simulink model "A17_PID_Lorentzaktuator"  (R2017b)
settings: Solver=ode45  StartTime=0.0  StopTime=15  MaxStep=1e-4  RelTol=1e-3  EnableMultiTasking=on
model workspace (MAT data in the model file):
  CF = 200000
  CR = 10
  KF = 50
  KV = 50
  LM = 0.01
  RM = 4
  Umax = 120
  g = 9.81
  m1 = 1
  m2 = 4
values from neighbouring files (symbols this model uses):
  CD = 1e1    (= 10)    [A14_Konstanten.m]    (also in A17_Konstanten.m = 100; A8_Konstanten.m = 20; A9_Konstanten.m = 0.1)
undefined symbols (not defined in the file or in its folder): sigbuilder_block
libraries: simulink x3
settings Model: Creator=jbaur  LastModifiedBy=jbaur
settings DataIOCC: ExternalInput=X1  SaveFormat=StructureWithTime  InspectSignalLogs=on  SignalLoggingName=sigsOut
settings OptimizationCC: ExpressionDepthLimit=2147483647  InitFltsAndDblsToZero=on  LifeSpan=inf
settings DebuggingCC: SaveWithParameterizedLinksMsg=none  SignalResolutionControl=TryResolveAllWithWarning  MultiTaskDSMMsg=warning  MultiTaskCondExecSysMsg=none  StateNameClashWarn=warning  SFUnexpectedBacktrackingDiag=warning  SFNoUnconditionalDefaultTransitionDiag=warning  SFExecutionAtInitializationDiag=none
settings HardwareCC: ProdBitPerPointer=32  ProdBitPerSizeT=32  ProdBitPerPtrDiffT=32  ProdLargestAtomicFloat=None  ProdIntDivRoundTo=Undefined  ProdEndianess=Unspecified  ProdWordSize=32  ProdHWDeviceType=32-bit Generic  TargetUnknown=on
settings ModelReferenceCC: PropagateSignalLabelsOutOfModel=off
settings CodeAppCC: StateflowObjectComments=on
settings GRTTargetCC: TargetFcnLib=ansi_tfl_tmw.mat  TargetLangStandard=C89/C90 (ANSI)  ModelReferenceCompliant=off  GeneratePreprocessorConditionals=Disable all  CombineOutputUpdateFcns=off  MatFileLogging=off  GRTInterface=on
settings ConfigComp: CovMetricSettings=dw  CovHtmlReporting=on  CovSaveCumulativeToWorkspaceVar=on  CovSaveSingleToWorkspaceVar=on  CovExternalEMLEnable=off  CovSFcnEnable=off

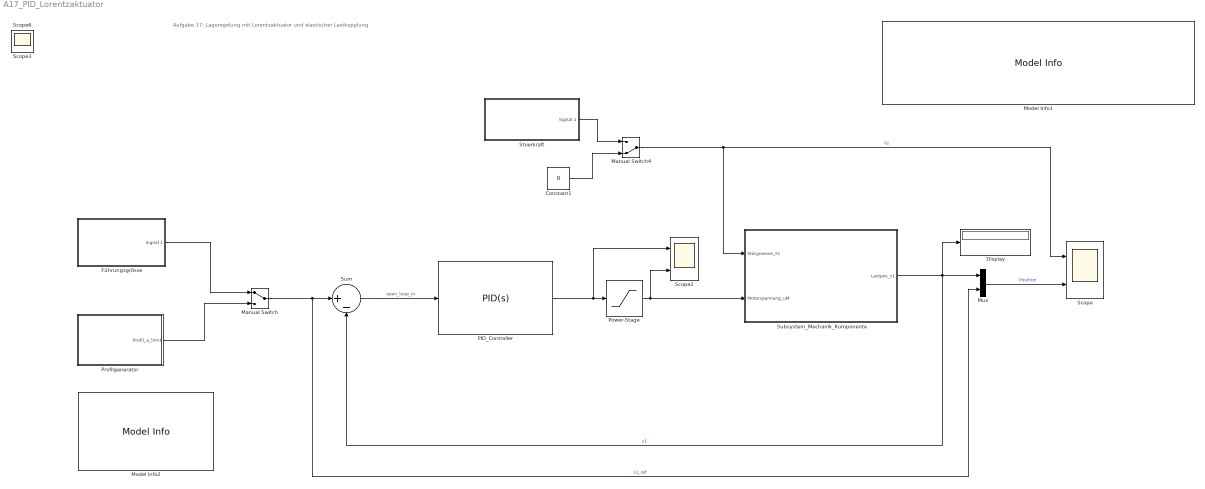
== system A17_PID_Lorentzaktuator ==
  note: Aufgabe 17: Lageregelung mit Lorentzaktuator und elastischer Lastkopplung
  Constant1 : Constant  Value=0
  Display : Display
  Führungsgrösse : Subsystem  Tag=STV Subsys  LoadFcn=sigbuilder_block('load');  StartFcn=sigbuilder_block('start');  StopFcn=sigbuilder_block('stop');  ClipboardFcn=sigbuilder_block('clipboard');  mask(Sigbuilder block){tuvar=[0:10]}
      mask help: Sigbuilder GUI
      mask init:
      | if ~strcmp(get_param(bdroot(gcbh),'SimulationStatus'),'stopped') tuvar = sigbuilder_block('maskInit'); end
      settings: CopyFcn=sigbuilder_block('copy');  DeleteFcn=sigbuilder_block('delete');  ModelCloseFcn=sigbuilder_block('modelClose');  PreSaveFcn=sigbuilder_block('preSave');  PauseFcn=sigbuilder_block('pause')  ContinueFcn=sigbuilder_block('continue')  NameChangeFcn=sigbuilder_block('namechange');  OpenFcn=sigbuilder_block('open',[221.25 181.5 954 508.5 ]);  CloseFcn=sigbuilder_block('close');
      mask Display: plot(0, 0, 100, 100,[2, 2, 32, 32, 2], [68, 8, 8, 68, 68],[32, 2], [38, 38], [32, 19, 2],[53, 60, 44], [32, 17, 17, 2],[16, 16, 31, 31]);txt = getActiveGroup(gcbh);text(2, 100, txt,'verticalAlignment', 'top');
  Manual Switch : ManualSwitch
  Manual Switch4 : ManualSwitch  CurrentSetting=0
  Model Info1 : simulink/Model-Wide Utilities/Model Info  Frame=on  DisplayStringWithTags=|  HorizontalTextAlignment=Left  LeftAlignmentValue=0.02
      | Motorparameter Maccon CFC90-HF-20
      | ----------------------------------------------------
      | UN=120V, Imax=10A
      | Fmax=500N, KF=50 N/A, RM=4Ohm, LM=10mH
      | max. Hub=20mm
  Model Info2 : simulink/Model-Wide Utilities/Model Info  Frame=on  DisplayStringWithTags=|  HorizontalTextAlignment=Left  LeftAlignmentValue=0.02
      | Bewegungsprofil:
      | ------------------------
      | smax = 0.1m
      | Tmax = 0.2s
      | amax = 10m/s^2
      | vmax = 1m/s
  Mux : Mux  Inputs=2
  PID_Controller : simulink/Continuous/PID Controller  Controller=PID  TimeDomain=Continuous-time  SampleTime=-1  IntegratorMethod=Forward Euler  FilterMethod=Forward Euler  Form=Ideal  UseFilter=on  ControllerParametersSource=internal  P=1000  I=0  D=0  N=100  InitialConditionSource=internal  InitialConditionForIntegrator=0  InitialConditionForFilter=0  ExternalReset=none  LimitOutput=off  UpperSaturationLimit=Umax  LowerSaturationLimit=-Umax  LinearizeAsGain=off  AntiWindupMode=clamping  Kb=1  TrackingMode=off  Kt=1  PParamMin=[]  PParamMax=[]  IParamMin=[]  IParamMax=[]  DParamMin=[]  DParamMax=[]  NParamMin=[]  NParamMax=[]  KbParamMin=[]  KbParamMax=[]  KtParamMin=[]  KtParamMax=[]  POutMin=[]  POutMax=[]  IOutMin=[]  IOutMax=[]  DOutMin=[]  DOutMax=[]  NOutMin=[]  NOutMax=[]  KbOutMin=[]  KbOutMax=[]  KtOutMin=[]  KtOutMax=[]  IntegratorOutMin=[]  IntegratorOutMax=[]  FilterOutMin=[]  FilterOutMax=[]  SumOutMin=[]  SumOutMax=[]  SumI1OutMin=[]  SumI1OutMax=[]  SumI2OutMin=[]  SumI2OutMax=[]  SumI3OutMin=[]  SumI3OutMax=[]  SumDOutMin=[]  SumDOutMax=[]  SaturationOutMin=[]  SaturationOutMax=[]  IntegratorContinuousStateAttributes=''  IntegratorStateMustResolveToSignalObject=off  IntegratorRTWStateStorageClass=Auto  FilterContinuousStateAttributes=''  FilterStateMustResolveToSignalObject=off  FilterRTWStateStorageClass=Auto  DifferentiatorICPrevScaledInput=0  DifferentiatorOutMin=[]  DifferentiatorOutMax=[]  InitialConditionSetting=State (most efficient)  FilterDiffOutCoefMin=[]  FilterDiffOutCoefMax=[]  SumDenOutMin=[]  SumDenOutMax=[]  SumNumOutMin=[]  SumNumOutMax=[]  ReciprocalOutMin=[]  ReciprocalOutMax=[]  DivideOutMin=[]  DivideOutMax=[]  TunerSelectOption=Transfer Function Based (PID Tuner App)
  Power-Stage : Saturate  UpperLimit=Umax  LowerLimit=-Umax
  Profilgenerator : Subsystem
  Scope : Scope  NumInputPorts=2
  Scope2 : Scope  NumInputPorts=2
  Stoerkraft : Subsystem  Tag=STV Subsys  LoadFcn=sigbuilder_block('load');  StartFcn=sigbuilder_block('start');  StopFcn=sigbuilder_block('stop');  ClipboardFcn=sigbuilder_block('clipboard');  mask(Sigbuilder block){tuvar=[0:10]}
      mask help: Sigbuilder GUI
      mask init:
      | if ~strcmp(get_param(bdroot(gcbh),'SimulationStatus'),'stopped') tuvar = sigbuilder_block('maskInit'); end
      settings: CopyFcn=sigbuilder_block('copy');  DeleteFcn=sigbuilder_block('delete');  ModelCloseFcn=sigbuilder_block('modelClose');  PreSaveFcn=sigbuilder_block('preSave');  PauseFcn=sigbuilder_block('pause')  ContinueFcn=sigbuilder_block('continue')  NameChangeFcn=sigbuilder_block('namechange');  OpenFcn=sigbuilder_block('open',[4.5 27.75 954 508.5 ]);  CloseFcn=sigbuilder_block('close');
      mask Display: plot(0, 0, 100, 100,[2, 2, 32, 32, 2], [68, 8, 8, 68, 68],[32, 2], [38, 38], [32, 19, 2],[53, 60, 44], [32, 17, 17, 2],[16, 16, 31, 31]);txt = getActiveGroup(gcbh);text(2, 100, txt,'verticalAlignment', 'top');
  Subsystem_Mechanik_Komponente : Subsystem
  Sum : Sum  Inputs=|+-
  Scope3 : Scope
  Scope6 : Scope
  wires:
  Sum/1 -> PID_Controller/1  "open_loop_in"
  PID_Controller/1 -> Scope2/1, Power-Stage/1
  Stoerkraft/1(Signal 1) -> Manual Switch4/1
  Constant1/1 -> Manual Switch4/2
  Manual Switch4/1 -> Subsystem_Mechanik_Komponente/1(Störgroesse_Fz), Scope/1  "Fz"
  Mux/1 -> Scope/2  "Position"
  Subsystem_Mechanik_Komponente/1(Lastpos_s1) -> Display/1, Mux/1, Sum/2  "s1"
  Manual Switch/1 -> Mux/2, Sum/1  "s1_ref"
  Profilgenerator/1(Profil_a_limit) -> Manual Switch/2
  Führungsgrösse/1(Signal 1) -> Manual Switch/1
  Power-Stage/1 -> Subsystem_Mechanik_Komponente/2(Motorspannung_uM), Scope2/2

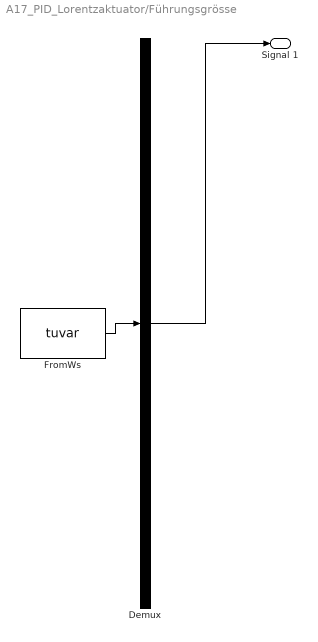
== system A17_PID_Lorentzaktuator/Führungsgrösse ==
  Demux : Demux  Tag=STV Demux  Outputs=1
  FromWs : FromWorkspace  Tag=STV FromWs  VariableName=tuvar  SampleTime=0
      SigBuilderData=|
      | common.afterFinalStr = 'Extrapolate'
      | common.sampleTime = 0
      | dataSet.timeRange = [0 15]
      | dataSet.name = 'Group 1'
      | sbobj.Groups.Name = 'Group 1'
      | sbobj.Groups.Signals.Name = 'Signal 1'
      | sbobj.Groups.Signals.XData = [0 4 4 8 8 12 12 15]
      | sbobj.Groups.Signals.YData = [0 0 0.1 0.1 0.2 0.2 0 0]
      | sbobj.Groups.TimeRange = [0 15]
  Signal 1 : Outport  Tag=STV Outport
  wires:
  Demux/1 -> Signal 1/1
  FromWs/1 -> Demux/1

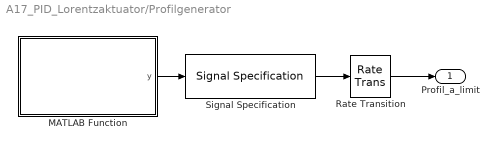
== system A17_PID_Lorentzaktuator/Profilgenerator ==
  MATLAB Function : MATLAB Function  TreatAsAtomicUnit=on
  Rate Transition : RateTransition
  Signal Specification : SignalSpecification  SampleTime=1e-4
  Profil_a_limit : Outport
  wires:
  Signal Specification/1 -> Rate Transition/1
  MATLAB Function/1(y) -> Signal Specification/1
  Rate Transition/1 -> Profil_a_limit/1

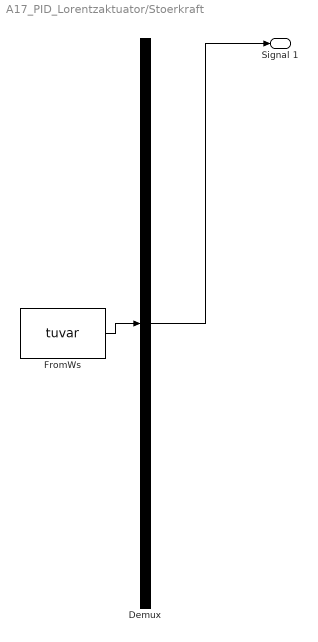
== system A17_PID_Lorentzaktuator/Stoerkraft ==
  Demux : Demux  Tag=STV Demux  Outputs=1
  FromWs : FromWorkspace  Tag=STV FromWs  VariableName=tuvar  SampleTime=0
      SigBuilderData=|
      | common.afterFinalStr = 'Extrapolate'
      | common.sampleTime = 0
      | dataSet.timeRange = [0 20]
      | dataSet.name = 'Group 1'
      | sbobj.Groups.Name = 'Group 1'
      | sbobj.Groups.Signals.Name = 'Signal 1'
      | sbobj.Groups.Signals.XData = [0 6 6 7 7 9 9 11 11 20]
      | sbobj.Groups.Signals.YData = [0 0 40 40 0 0 -40 -40 0 0]
      | sbobj.Groups.TimeRange = [0 20]
  Signal 1 : Outport  Tag=STV Outport
  wires:
  Demux/1 -> Signal 1/1
  FromWs/1 -> Demux/1

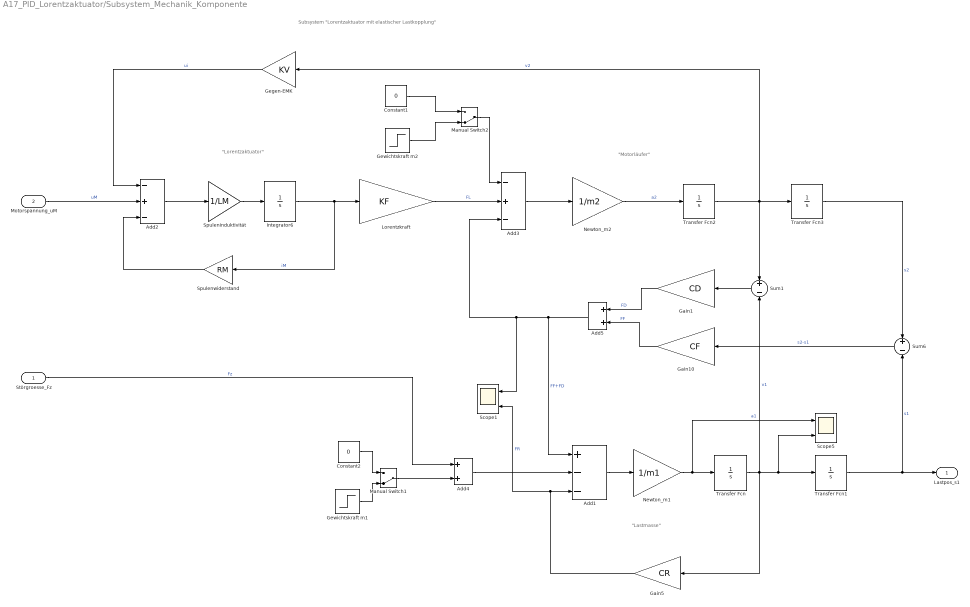
== system A17_PID_Lorentzaktuator/Subsystem_Mechanik_Komponente ==
  note: Subsystem "Lorentzaktuator mit elastischer Lastkopplung"
  note: "Motorläufer"
  note: "Lastmasse"
  note: "Lorentzaktuator"
  Störgroesse_Fz : Inport
  Motorspannung_uM : Inport  Port=2
  Add1 : Sum  Inputs=+--
  Add2 : Sum  Inputs=-+-
  Add3 : Sum  Inputs=-+-
  Add4 : Sum
  Add5 : Sum
  Constant1 : Constant  Value=0
  Constant2 : Constant  Value=0
  Gain1 : Gain  Gain=CD
  Gain10 : Gain  Gain=CF
  Gain5 : Gain  Gain=CR
  Gegen-EMK : Gain  Gain=KV
  Gewichtskraft m1 : Step  Time=0  After=m1*g  SampleTime=0
  Gewichtskraft m2 : Step  Time=0  After=m2*g  SampleTime=0
  Integrator6 : Integrator
  Lorentzkraft : Gain  Gain=KF
  Manual Switch1 : ManualSwitch  CurrentSetting=0
  Manual Switch2 : ManualSwitch  CurrentSetting=0
  Newton_m1 : Gain  Gain=1/m1
  Newton_m2 : Gain  Gain=1/m2
  Scope1 : Scope  NumInputPorts=2
  Scope5 : Scope  NumInputPorts=2
  Spuleninduktivität : Gain  Gain=1/LM
  Spulenwiderstand : Gain  Gain=RM
  Sum1 : Sum  Inputs=+|-
  Sum6 : Sum  Inputs=+|-
  Transfer Fcn{,1..3} (4 alike) : TransferFcn  Denominator=[1 0]
  Lastpos_s1 : Outport
  wires:
  Constant1/1 -> Manual Switch2/1
  Gewichtskraft m2/1 -> Manual Switch2/2
  Transfer Fcn2/1 -> Transfer Fcn3/1, Gegen-EMK/1, Sum1/1  "v2"
  Newton_m2/1 -> Transfer Fcn2/1  "a2"
  Sum6/1 -> Gain10/1  "s2-s1"
  Add5/1 -> Add1/1, Scope1/1, Add3/3  "FF+FD"
  Add1/1 -> Newton_m1/1
  Newton_m1/1 -> Transfer Fcn/1, Scope5/1  "a1"
  Gain5/1 -> Scope1/2, Add1/3  "FR"
  Lorentzkraft/1 -> Add3/2  "FL"
  Manual Switch2/1 -> Add3/1
  Add3/1 -> Newton_m2/1
  Transfer Fcn3/1 -> Sum6/1  "s2"
  Constant2/1 -> Manual Switch1/1
  Gewichtskraft m1/1 -> Manual Switch1/2
  Transfer Fcn/1 -> Transfer Fcn1/1, Scope5/2, Gain5/1, Sum1/2  "v1"
  Transfer Fcn1/1 -> Lastpos_s1/1, Sum6/2  "s1"
  Integrator6/1 -> Lorentzkraft/1, Spulenwiderstand/1  "iM"
  Spuleninduktivität/1 -> Integrator6/1
  Add2/1 -> Spuleninduktivität/1
  Spulenwiderstand/1 -> Add2/3
  Motorspannung_uM/1 -> Add2/2  "uM"
  Gegen-EMK/1 -> Add2/1  "ui"
  Störgroesse_Fz/1 -> Add4/1  "Fz"
  Manual Switch1/1 -> Add4/2
  Add4/1 -> Add1/2
  Sum1/1 -> Gain1/1
  Gain1/1 -> Add5/1  "FD"
  Gain10/1 -> Add5/2  "FF"

== matlab function A17_PID_Lorentzaktuator/Profilgenerator/MATLAB Function ==
  data: y output
function y = Zeitfunktion

% Deklaration der lokalen Variablen
Timestep = 1e-4;

% Deklaration der persistenten Zeitvariablen
persistent t

% Definition der Zeitfunktion
if isempty(t)
    t=0;
  else
    t = t + Timestep;
end

% Beschleunigungsbegrenztes Bewegungsprofil
s1_max = 0.1;
s2_max = 0.2;
s3_max = 0.2;
T1_max = 0.2;
T2_max = 0.2;
T3_max = 0.2;
t1 = T1_max/2;
t2 = T2_max/2;
t3 = T3_max/2;
a1_max = s1_max/t1^2;
a2_max = (s2_max-s1_max)/t2^2;
a3_max = s3_max/t3^2;
v1_max = a1_max*t1;
v2_max = a2_max*t2;
v3_max = a3_max*t3;

% Bereichsunterscheidung
if t<=4
    y = 0;
elseif (t>4 && t<=4+t1)
    y = 0.5*a1_max*(t-4)^2;
elseif (t>4+t1 && t<=4+T1_max)
    y = 0.5*s1_max + v1_max*(t-4-t1) - 0.5*a1_max*(t-4-t1)^2;
elseif (t>4+T1_max && t<=8)
    y = s1_max;
elseif (t>8 && t<=8+t2)
    y = s1_max + 0.5*a2_max*(t-8)^2;
elseif (t>8+t2 && t<=8+T2_max)
    y = s1_max + 0.5*(s2_max-s1_max) + v2_max*(t-8-t2) - 0.5*a2_max*(t-8-t2)^2;
elseif (t>8+T2_max && t<=12)
    y = s2_max;
elseif (t>12 && t<=12+t3)
    y = s3_max - 0.5*a3_max*(t-12)^2;
elseif (t>12+t3 && t<=12+T3_max)
    y = s3_max - (0.5*s3_max + v3_max*(t-12-t3) - 0.5*a3_max*(t-12-t3)^2);
else
    y = 0;
end
